simulink model "Day17"  (R2024b)
settings: Solver=VariableStepAuto  StartTime=0.0  StopTime=10.0  RelTol=1e-3
settings Model: Creator=jun_mac  LastModifiedBy=jun_mac

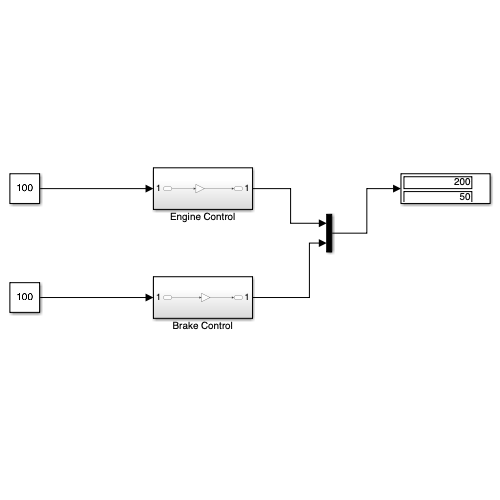
[thumbnail: Simulink's stored preview of the top-level diagram]
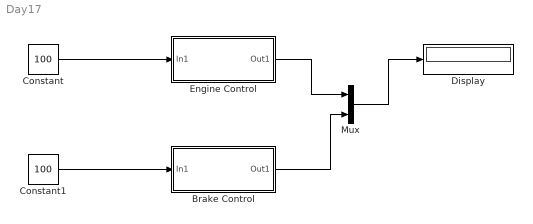
== system Day17 ==
  Brake Control : Subsystem
  Constant : Constant  Value=100
  Constant1 : Constant  Value=100
  Display : Display
  Engine Control : Subsystem
  Mux : Mux  Inputs=2
  wires:
  Constant/1 -> Engine Control/1(In1)
  Engine Control/1(Out1) -> Mux/1
  Brake Control/1(Out1) -> Mux/2
  Mux/1 -> Display/1
  Constant1/1 -> Brake Control/1(In1)

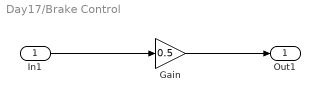
== system Day17/Brake Control ==
  In1 : Inport
  Gain : Gain  Gain=0.5
  Out1 : Outport
  wires:
  In1/1 -> Gain/1
  Gain/1 -> Out1/1

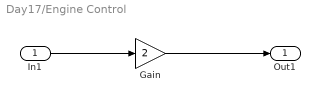
== system Day17/Engine Control ==
  In1 : Inport
  Gain : Gain  Gain=2
  Out1 : Outport
  wires:
  In1/1 -> Gain/1
  Gain/1 -> Out1/1
